simulink model "questA_initial_model"  (R2018a)
settings: Solver=VariableStepAuto  StartTime=0.0  StopTime=8.0  RelTol=1e-3
values from neighbouring files (symbols this model uses):
  A = [0 1 0 0; 20.6 0 0 0; 0 0 0 1; -.5 0 0 0]    [InvertedPendulum.m]
  B = [0; -1; 0; .5]    [InvertedPendulum.m]
  C = [1 0 0 0; 0 0 1 0]    [InvertedPendulum.m]
  x0 = [-.2; -.06; .01; .3]    [InvertedPendulum.m]
settings Model: Creator=Administrator  LastModifiedBy=Administrator

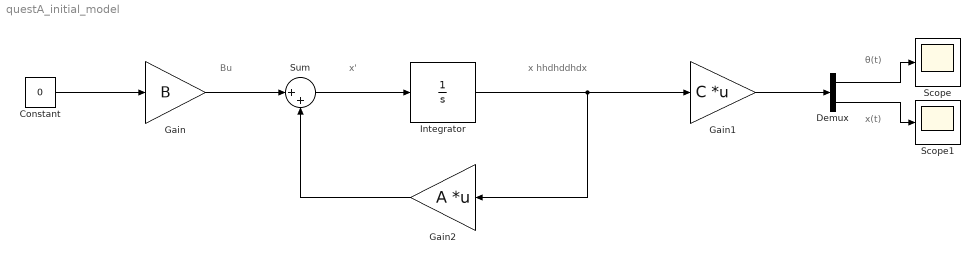
== system questA_initial_model ==
  note: x(t)
  note: θ(t)
  note: Bu
  note: x'
  note: x
      |
      | hhdhddhdx
  Constant : Constant  Value=0
  Demux : Demux  Outputs=2
  Gain : Gain  Gain=B
  Gain1 : Gain  Gain=C  Multiplication=Matrix(K*u)
  Gain2 : Gain  Gain=A  Multiplication=Matrix(K*u)
  Integrator : Integrator  InitialCondition=x0
  Scope : Scope
  Scope1 : Scope
  Sum : Sum  Inputs=|++
  wires:
  Gain/1 -> Sum/1
  Sum/1 -> Integrator/1
  Integrator/1 -> Gain1/1, Gain2/1
  Gain1/1 -> Demux/1
  Gain2/1 -> Sum/2
  Constant/1 -> Gain/1
  Demux/1 -> Scope/1
  Demux/2 -> Scope1/1
